simulink model "sep_rover_full"  (R2024b)
settings: Solver=FixedStepDiscrete  StartTime=0  StopTime=300  FixedStep=0.0005  RelTol=1e-3
settings Model: SimulationMode=accelerator  Creator=Usuario  LastModifiedBy=Usuario

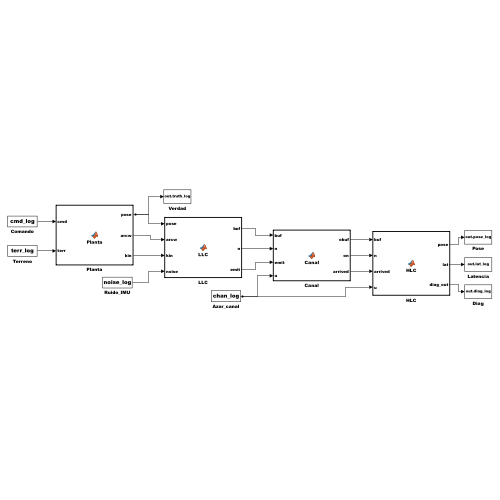
[thumbnail: Simulink's stored preview of the top-level diagram]
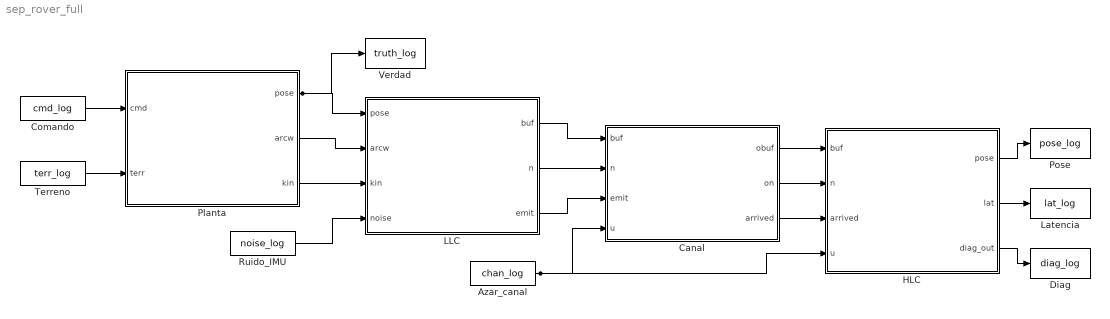
== system sep_rover_full ==
  Azar_canal : FromWorkspace  VariableName=chan_log  SampleTime=0.0005  Interpolate=off  OutputAfterFinalValue=Holding final value
  Canal : MATLAB Function  TreatAsAtomicUnit=on
  Comando : FromWorkspace  VariableName=cmd_log  SampleTime=0.0005  Interpolate=off  OutputAfterFinalValue=Holding final value
  Diag : ToWorkspace  VariableName=diag_log  SaveFormat=Timeseries  SampleTime=0.0005
  HLC : MATLAB Function  TreatAsAtomicUnit=on
  LLC : MATLAB Function  TreatAsAtomicUnit=on
  Latencia : ToWorkspace  VariableName=lat_log  SaveFormat=Timeseries  SampleTime=0.0005
  Planta : MATLAB Function  TreatAsAtomicUnit=on
  Pose : ToWorkspace  VariableName=pose_log  SaveFormat=Timeseries  SampleTime=0.0005
  Ruido_IMU : FromWorkspace  VariableName=noise_log  SampleTime=0.0005  Interpolate=off  OutputAfterFinalValue=Holding final value
  Terreno : FromWorkspace  VariableName=terr_log  SampleTime=0.0005  Interpolate=off  OutputAfterFinalValue=Holding final value
  Verdad : ToWorkspace  VariableName=truth_log  SaveFormat=Timeseries  SampleTime=0.0005
  wires:
  Comando/1 -> Planta/1(cmd)
  Azar_canal/1 -> HLC/4(u), Canal/4(u)
  Terreno/1 -> Planta/2(terr)
  Ruido_IMU/1 -> LLC/4(noise)
  Planta/1(pose) -> LLC/1(pose), Verdad/1
  Planta/3(kin) -> LLC/3(kin)
  Planta/2(arcw) -> LLC/2(arcw)
  LLC/1(buf) -> Canal/1(buf)
  LLC/2(n) -> Canal/2(n)
  LLC/3(emit) -> Canal/3(emit)
  Canal/1(obuf) -> HLC/1(buf)
  Canal/2(on) -> HLC/2(n)
  Canal/3(arrived) -> HLC/3(arrived)
  HLC/1(pose) -> Pose/1
  HLC/2(lat) -> Latencia/1
  HLC/3(diag_out) -> Diag/1

== matlab function sep_rover_full/LLC ==
  data: pose input; buf output; arcw input; kin input; noise input; n output; emit output
function [buf, n, emit] = LLC(pose, arcw, kin, noise)
persistent st sp lp gp
if isempty(st)
    sp = sim_params(); lp = llc_params(); gp = sep_geo_params();
    st = llc_init();
end
buf = zeros(1, raw_buf_max(), 'uint8'); n = 0; emit = false;
[st, b, nn, e] = llc_step(st, kin(1), kin(2:3), kin(4), kin(5), arcw, ...
                          noise, lp, gp, sp.imu, sp.sim.Tb);
buf(:) = b; n = nn; emit = e;
end

== matlab function sep_rover_full/Planta ==
  data: cmd input; pose output; terr input; arcw output; kin output
function [pose, arcw, kin] = Planta(cmd, terr)
persistent st sp
if isempty(st)
    sp = sim_params();
    st = plant_init();
end
pose = zeros(1,3); arcw = zeros(1,6); kin = zeros(1,5);
[st, o] = plant_step(st, cmd(1), cmd(2), terr(3:8), terr(1), terr(2), ...
                     sp.sim.Tb, sp.plant);
pose(:) = o.pose;
arcw(:) = o.arc;
kin(:)  = [o.w, o.a_body, terr(1), terr(2)];
end

== matlab function sep_rover_full/Canal ==
  data: buf input; n input; emit input; u input; obuf output; on output; arrived output
function [obuf, on, arrived] = Canal(buf, n, emit, u)
persistent st sp
if isempty(st)
    sp = sim_params();
    st = channel_init(sp.chan);
end
obuf = zeros(1, raw_buf_max(), 'uint8'); on = 0; arrived = false;
[st, b, nn, a] = channel_step(st, buf, n, emit, u, sp.chan, sp.sim.Tb);
obuf(:) = b; on = nn; arrived = a;
end

== matlab function sep_rover_full/HLC ==
  data: buf input; n input; arrived input; u input; pose output; lat output; diag_out output
function [pose, lat, diag_out] = HLC(buf, n, arrived, u)
persistent st sp gp ep
if isempty(st)
    sp = sim_params(); gp = sep_geo_params(); ep = sep_ekf_params();
    st = hlc_init(ep);
end
pose = zeros(5,1); lat = 0; diag_out = zeros(3,1);
[st, x, ~, dg, l, ~] = hlc_step(st, buf, n, arrived, ...
                                gp, ep, sp.agents, sp.sim.Tb, u(3));
pose(:) = x; diag_out(:) = dg; lat = l;
end
